simulink model "MNIST_2level_NN_4_2"  (R2015b)
settings: Solver=VariableStepAuto  StartTime=0.0  StopTime=10.0  RelTol=1e-3
libraries: neural x13
(part 2 of 3)

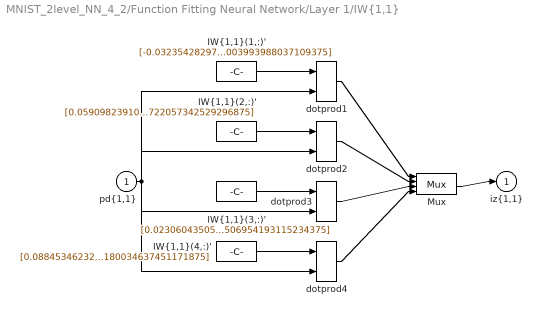
== system MNIST_2level_NN_4_2/Function Fitting Neural Network/Layer 1/IW{1,1} ==
  "pd{1,1}" : Inport  PortDimensions=717
      mask Display: e = 0.06;c1 = [120 230 180]/255;c2 = ([120 230 180]+0)/(256+128);c3 = ([120 230 180]+128)/(256+128);patch([0 1 1 0],[0 0 1 1],c1);patch([0 1 1 1-e 1-e 0+e],[0 0 1 1-e 0+e 0+e],c2);patch([0 0 1 1-e 0+e 0+e],[0 1 1 1-e 1-e 0+e],c3);plot([0 1 1 0 0],[0 0 1 1 0]);
  "IW{1,1}(1,:)'" : Constant  Value=[-0.03235428297048294210558339045746834017336368560791015625;0.0103274441299610331146396902113338001072406768798828125;0.0176947566460041762204102866462562815286219120025634765625;0.01481901960590031701314739365216155420057475566864013671875;-0.05346805921825574514638645950981299392879009246826171875;0.0211052936800935168892845439359007286839187145233154296875;-0.0276538972098966141788256578593063750304281711578369140625;-0.07238146656643036636058496924306382425129413604736328125;0.02309372950761180709466913185679004527628421783447265625;0.0138971869634534651860580112270326935686171054840087890625;0.070541532563377362663459280156530439853668212890625;0.0305734448181651796705438073331606574356555938720703125;0.055097744907471823960776191597688011825084686279296875;-0.0801840844261189344965856662383885122835636138916015625;0.041891774188532716893806906455210992135107517242431640625;-0.0732924240655477843287002315264544449746608734130859375;-0.04545803202608462989520177188751404173672199249267578125;0.0634378332510132925126100644774851389229297637939453125;-0.025094974420825831573633735160910873673856258392333984375;0.00904411601716214978707863991758131305687129497528076171875;0.0105876784212682283070616762188365100882947444915771484375;-0.07024624073187575590271336523073841817677021026611328125;-0.075132490839150134487312016062787733972072601318359375;0.019137995736216939501872502660262398421764373779296875;-0.06505414799649540669168601425553788430988788604736328125;-0.01031884970695987925604075741148335509933531284332275390625;-0.084894712689648599290848096643458120524883270263671875;0.042870409751250664054378347600504639558494091033935546875;-0.060059362195281552898595833767103613354265689849853515625;-0.07512266961269127574229997890142840333282947540283203125;0.0512760806485703934942677051367354579269886016845703125;0.048783902609691336127450966841934132389724254608154296875;-0.033173678679507441480200924388554994948208332061767578125;-0.072945991231301743340509347035549581050872802734375;0.05793340649779017692555527219155919738113880157470703125;-0.04486774167644301536395090579389943741261959075927734375;0.04161382223009717218342728983770939521491527557373046875;-0.07017481158577086597372129972427501343190670013427734375;0.02310481342603522281198280552416690625250339508056640625;0.0864315721094397748647253365561482496559619903564453125;0.059155332248012892915056681886198930442333221435546875;0.037572637167272271430107366541051305830478668212890625;0.042868845706902240777491641665619681589305400848388671875;0.04851794939651166149729988319450058043003082275390625;-0.01317815460740855322552267381297497195191681385040283203125;-0.0113293834130685742989097519739516428671777248382568359375;0.009091744050230977924886843766216770745813846588134765625;-0.046491015794172863007105434007826261222362518310546875;0.0032601681138438622087338814026225009001791477203369140625;-0.022764559347166805902684671991664799861609935760498046875;-0.0654001104514720932314730816869996488094329833984375;-0.05728135306754240929638655188682605512440204620361328125;0.0399575173854561926933826043750741519033908843994140625;-0.06728199884128048535725241663385531865060329437255859375;0.00427302389499006028683592006700564525090157985687255859375;-0.049462127823360936551555511186961666680872440338134765625;-0.09090426786975937256674029640635126270353794097900390625;0.06302530590246670227916325757178128696978092193603515625;-0.06266910791830075655450826843662071041762828826904296875;-0.0127530962626631015621736509046968421898782253265380859375;0.0145386640548171540421318326252730912528932094573974609375;-0.09393657504801122826165737933479249477386474609375;-0.04813019827135779638016543913181521929800510406494140625;-0.02943971723029285836314983271222445182502269744873046875;0.015073182812351072767942383734407485462725162506103515625;0.118462792713101616737247923083486966788768768310546875;-0.054802237546599907869193657461437396705150604248046875 ...(+38052 chars)]
      mask Display: e = 0.06;c1 = [120 150 230]/255;c2 = ([120 150 230]+0)/383;c3 = ([120 150 230]+128)/383;patch([0 1 1 0],[0 0 1 1],c1);patch([0 1 1 1-e 1-e 0+e],[0 0 1 1-e 0+e 0+e],c2);patch([0 0 1 1-e 0+e 0+e],[0 1 1 1-e 1-e 0+e],c3);plot([0 1 1 0 0],[0 0 1 1 0]);disp('Weights');
  "IW{1,1}(2,:)'" : Constant  Value=[0.05909823910424101545135755486626294441521167755126953125;-0.11063877768862225015045197551444289274513721466064453125;0.0271832782062883804297115375447901897132396697998046875;-0.0859657250700465447312836886339937336742877960205078125;-0.10996227396293412059691263493732549250125885009765625;-0.05774570732365759406778948914507054723799228668212890625;-0.04597012975111337829137170274407253600656986236572265625;-0.025176179926081447557617565280452254228293895721435546875;0.025926962557053574720544730780602549202740192413330078125;-0.0882474243169806549236255932555650360882282257080078125;-0.051678015585380633611922718273490318097174167633056640625;-0.0704386619931114399406624215771444141864776611328125;0.06497320986555045474464264998459839262068271636962890625;-0.07038514701655163019466954210656695067882537841796875;-0.07273877494510046226583455108993803150951862335205078125;-0.0714381147105269953545558792029623873531818389892578125;0.0402601596472166589624208654640824533998966217041015625;-0.05990407934523755972833214400452561676502227783203125;-0.00839637742917633510264519003385430551134049892425537109375;0.03227935669884916813909825350492610596120357513427734375;-0.023274352039388164492539345928889815695583820343017578125;0.03952540793766191884461846939302631653845310211181640625;-0.0025850109436221964387403460250425268895924091339111328125;0.02469038437799207785783295321380137465894222259521484375;0.056488009192813048997550140484236180782318115234375;0.07085741244594088994457337093990645371377468109130859375;0.064346185284777590585036932679940946400165557861328125;0.047844163446901920300202704083858407102525234222412109375;0.0346756208637023222163264790651737712323665618896484375;-0.06971317788310767149528857089535449631512165069580078125;-0.0076965423623347357928725642750578117556869983673095703125;0.0002632085916607039555170644007375813089311122894287109375;-0.1049885487833850661321122288427432067692279815673828125;-0.0736637458040042270024372328407480381429195404052734375;0.060951124486899176113663401110898121260106563568115234375;0.054711889777745430218924838072780403308570384979248046875;-0.05139380029613634104368458110911888070404529571533203125;-0.1065151522108815085321253945949138142168521881103515625;-0.11277076895895309094353109458097605966031551361083984375;-0.11301254120010183201738840352845727466046810150146484375;0.02940084647104986015353489392509800381958484649658203125;-0.04335946767419705805135521359261474572122097015380859375;-0.0637973256770569541185267326000030152499675750732421875;-0.0967150461675463091193449827187578193843364715576171875;-0.0335001703757568380925846440732129849493503570556640625;-0.0193125988990643128462298960812404402531683444976806640625;-0.05277626824666113714012993796131922863423824310302734375;0.05206563878695201486035415427977568469941616058349609375;-0.0106732116198309280596934200957548455335199832916259765625;-0.07332997457257857398804645754353259690105915069580078125;-0.059960814111750693200519890524446964263916015625;0.08506802150818042196345203365126508288085460662841796875;0.0955809832640759082789116973799536935985088348388671875;-0.032717683407469992651339651956732268445193767547607421875;0.016131065543820495566951223054275033064186573028564453125;-0.06227822187022613587004116197931580245494842529296875;-0.06846433328023730779943178959001670591533184051513671875;0.0230072126782046061654884994140957132913172245025634765625;-0.032577027735492224136404360024243942461907863616943359375;-0.07628632721471755029352124211072805337607860565185546875;-0.053783031611663388582567080220542266033589839935302734375;0.02025680437429579205943497299813316203653812408447265625;-0.094796026953707979156860119474004022777080535888671875;0.01381880409777080931377213346422649919986724853515625;0.071265660360969540487730000677402131259441375732421875;-0.000460080279002857139847293410639395006000995635986328125;0.0288964728883088391164779551445462857373058795928955078125 ...(+38203 chars)]
      mask Display: e = 0.06;c1 = [120 150 230]/255;c2 = ([120 150 230]+0)/383;c3 = ([120 150 230]+128)/383;patch([0 1 1 0],[0 0 1 1],c1);patch([0 1 1 1-e 1-e 0+e],[0 0 1 1-e 0+e 0+e],c2);patch([0 0 1 1-e 0+e 0+e],[0 1 1 1-e 1-e 0+e],c3);plot([0 1 1 0 0],[0 0 1 1 0]);disp('Weights');
  "IW{1,1}(3,:)'" : Constant  Value=[0.0230604350500326800432748797220483538694679737091064453125;0.0332195632068573443174130943589261732995510101318359375;0.01823977961070107067786949528453988023102283477783203125;0.0126000590970618379926815322278343955986201763153076171875;-0.09556806792189169452722552478007855825126171112060546875;0.056153363253581257963364947727313847281038761138916015625;0.0212238743876330022974929789825182524509727954864501953125;-0.0343137154561568291644135797469061799347400665283203125;-0.0641979971225328238659812996047548949718475341796875;-0.0906030778203754660893309846869669854640960693359375;-0.005262978385187445928838911868297145701944828033447265625;-0.0235390507036290878850604002536783809773623943328857421875;-0.016398664096076341623042793571585207246243953704833984375;0.03598394526192995324098689025049679912626743316650390625;0.051911916684415922162987300225722719915211200714111328125;-0.013460443524568981021882763116082060150802135467529296875;-0.0186532887222654077119532445294680655933916568756103515625;0.02319669304613204696696726614391081966459751129150390625;-0.08694318144015132643342980145462206564843654632568359375;0.0722566410135369319167608637144439853727817535400390625;-0.101299396945041253470520814516930840909481048583984375;-0.053391410065484527780466095236988621763885021209716796875;-0.0658850548994747153841444742283783853054046630859375;-0.033517383900770615634545634975438588298857212066650390625;-0.08688951706567805965963913195082568563520908355712890625;-0.1056355156247527349311354782912530936300754547119140625;-0.110674341448736723858559116706601344048976898193359375;-0.09838640799246987922455076613914570771157741546630859375;-0.03758309357494836466795362639459199272096157073974609375;-0.09190894446234827708241965638080728240311145782470703125;-0.0168153895647655850231760865653996006585657596588134765625;-0.05143370594215614099997679886655532754957675933837890625;-0.071020599204288215045011156689724884927272796630859375;-0.039450419878958135899704728899450856260955333709716796875;-0.026708974792534319331327452573532355017960071563720703125;-0.0476535638845049513978580080220126546919345855712890625;-0.060163611467376150454544614376573008485138416290283203125;0.08897452209162474978665358094076509587466716766357421875;-0.026703665294301341670557548013675841502845287322998046875;-0.034560701713767467968541069467391935177147388458251953125;0.07013908276332965485710957409537513740360736846923828125;0.070048677745446263909201434216811321675777435302734375;-0.022393052106942930301602956433271174319088459014892578125;0.06641366179591734475451403341139666736125946044921875;-0.023326390456857644395416429006218095310032367706298828125;0.04073493833670484287612367779729538597166538238525390625;0.0272609649376160424749659938470358611084520816802978515625;0.038759543310952028483118425583597854711115360260009765625;-0.078972098571666704547311610440374352037906646728515625;0.026416398810247439243870104519373853690922260284423828125;-0.08325213289088850832087018716265447437763214111328125;-0.049035772839232265318809567133939708583056926727294921875;-0.053087074628186660396611529222354874946177005767822265625;-0.015122581482854231815782242165369098074734210968017578125;-0.07137007469602674181174961631768383085727691650390625;-0.03483293128367460911309905213784077204763889312744140625;0.0275187309490855964988487158962016110308468341827392578125;-0.0253042908169711054655603987839640467427670955657958984375;0.05996699735190909319459962034670752473175525665283203125;-0.0274887263657122467297444501355130341835319995880126953125;-0.03828407690606912272546225040059653110802173614501953125;0.086978383397274872113058563627419061958789825439453125;0.0304157287819946907381218892396645969711244106292724609375;-0.04571025059088883180091755775720230303704738616943359375;0.02811448319858424194084278724403702653944492340087890625;0.0734026946550236647492937436254578642547130584716796875;0.01918768359524940236848777885825256817042827606201171875 ...(+37999 chars)]
      mask Display: e = 0.06;c1 = [120 150 230]/255;c2 = ([120 150 230]+0)/383;c3 = ([120 150 230]+128)/383;patch([0 1 1 0],[0 0 1 1],c1);patch([0 1 1 1-e 1-e 0+e],[0 0 1 1-e 0+e 0+e],c2);patch([0 0 1 1-e 0+e 0+e],[0 1 1 1-e 1-e 0+e],c3);plot([0 1 1 0 0],[0 0 1 1 0]);disp('Weights');
  "IW{1,1}(4,:)'" : Constant  Value=[0.08845346232223338933664535943535156548023223876953125;0.08384236208057922745684464871374075300991535186767578125;-0.0145091735625332736436821079450965044088661670684814453125;-0.079904581545591268909589643953950144350528717041015625;0.06281834868389786497022697631109622307121753692626953125;-0.0793864400160162186903534120574477128684520721435546875;0.058545212196975761342887523142053396441042423248291015625;0.031560198536786245038232578963288688100874423980712890625;0.03746076200861032934330552279789117164909839630126953125;0.004079847077972977194282311330653101322241127490997314453125;-0.0449187477375685706437735689178225584328174591064453125;0.04110163401391146720253999546912382356822490692138671875;-0.06009990754568415860514818405135883949697017669677734375;-0.039185139164148126422748674713147920556366443634033203125;-0.0219918000224269272191435220520361326634883880615234375;0.00140104722012515496565310257892633671872317790985107421875;0.0154463697307633783528668658391325152479112148284912109375;0.04930750317667327575765767733173561282455921173095703125;-0.08231298093131873827577038582603563554584980010986328125;-0.07114865389620728119979276016238145530223846435546875;-0.0309649720783258912415458752320773783139884471893310546875;0.0063595110033314063147091843575253733433783054351806640625;0.032422398301778850016052757609941181726753711700439453125;-0.07017440293081970981159400935212033800780773162841796875;0.06403469575506580413470913981655030511319637298583984375;-0.003827312327512095817272363973415849613957107067108154296875;0.05424232994941939611788228603472816757857799530029296875;-0.0131154319776103610306616786829181364737451076507568359375;0.07973984327983629771807727593113668262958526611328125;-0.060175276416224006414967817590877530165016651153564453125;-0.059139066704392860562844447258612490259110927581787109375;0.0075054866431869537990451135556213557720184326171875;-0.0630145382175688606452013118541799485683441162109375;-0.07619383335451186678444202016180497594177722930908203125;0.0037356429186327223639085826079053731518797576427459716796875;-0.06527989083661576985573304909848957322537899017333984375;-0.012942874094519003780323629371196147985756397247314453125;0.08622546647598712532545306430620257742702960968017578125;-0.0275314724130845435434711276911912136711180210113525390625;-0.072911342779214016740496617785538546741008758544921875;-0.02746065005392651914295498727369704283773899078369140625;-0.07313951242317895395927962454152293503284454345703125;0.0153775764054662443525156589885227731429040431976318359375;0.049219879472240123108317533251465647481381893157958984375;-0.03314701592432862942150251228667912073433399200439453125;0.05600025147720071039270095525353099219501018524169921875;0.0112276901319347428842565506101891514845192432403564453125;0.015372198393586104792074564784343237988650798797607421875;-0.0289011683761912392676141081437890534289181232452392578125;-0.049881973166923172791076268595134024508297443389892578125;-0.01254350204826501676003136509507385198958218097686767578125;-0.060285525106897226710334081190012511797249317169189453125;-0.06797151126091606487822360804784693755209445953369140625;-0.0363057279877211092067312847575522027909755706787109375;-0.064215961796205422995598155466723255813121795654296875;0.004586956694110169187317271877191160456277430057525634765625;-0.07941236194212207555320759411188191734254360198974609375;0.01957736770554845129321819285905803553760051727294921875;0.013893918841882159365130888772910111583769321441650390625;0.027834993732121886267361077216264675371348857879638671875;0.09238437159152006195039774638644303195178508758544921875;0.056406981122189787936083149588739615865051746368408203125;0.030658690560729943974660471894821966998279094696044921875;0.014764924428758881280732140339750912971794605255126953125;0.05688955225242715851852182140646618790924549102783203125;-0.0703582569179704020445598189326119609177112579345703125 ...(+38310 chars)]
      mask Display: e = 0.06;c1 = [120 150 230]/255;c2 = ([120 150 230]+0)/383;c3 = ([120 150 230]+128)/383;patch([0 1 1 0],[0 0 1 1],c1);patch([0 1 1 1-e 1-e 0+e],[0 0 1 1-e 0+e 0+e],c2);patch([0 0 1 1-e 0+e 0+e],[0 1 1 1-e 1-e 0+e],c3);plot([0 1 1 0 0],[0 0 1 1 0]);disp('Weights');
  Mux : Mux
      mask Display: e = 0.06;c1 = [120 150 230]/255;c2 = ([120 150 230]+0)/383;c3 = ([120 150 230]+128)/383;patch([0 1 1 0],[0 0 1 1],c1);patch([0 1 1 1-e 1-e 0+e],[0 0 1 1-e 0+e 0+e],c2);patch([0 0 1 1-e 0+e 0+e],[0 1 1 1-e 1-e 0+e],c3);plot([0 1 1 0 0],[0 0 1 1 0]);disp('Mux');
  dotprod{1..4} (4 alike) : neural/Weight Functions/dotprod
  "iz{1,1}" : Outport
      mask Display: e = 0.06;c1 = [120 230 180]/255;c2 = ([120 230 180]+0)/(256+128);c3 = ([120 230 180]+128)/(256+128);patch([0 1 1 0],[0 0 1 1],c1);patch([0 1 1 1-e 1-e 0+e],[0 0 1 1-e 0+e 0+e],c2);patch([0 0 1 1-e 0+e 0+e],[0 1 1 1-e 1-e 0+e],c3);plot([0 1 1 0 0],[0 0 1 1 0]);
  wires:
  "IW{1,1}(1,:)'"/1 -> dotprod1/1
  "pd{1,1}"/1 -> dotprod1/2, dotprod2/2, dotprod3/2, dotprod4/2
  dotprod1/1 -> Mux/1
  "IW{1,1}(2,:)'"/1 -> dotprod2/1
  dotprod2/1 -> Mux/2
  "IW{1,1}(3,:)'"/1 -> dotprod3/1
  dotprod3/1 -> Mux/3
  "IW{1,1}(4,:)'"/1 -> dotprod4/1
  dotprod4/1 -> Mux/4
  Mux/1 -> "iz{1,1}"/1
